simulink model "SecRwLtStHdrstFwdBkwdIsPosChk"  (R2024b)
settings: Solver=FixedStepDiscrete  StartTime=0.0  StopTime=10.0  FixedStep=0.01  RelTol=1e-3
undefined symbols (not defined in the file or in its folder): KeSMSuSecRwStHeadrestFwdBkwdPosDelta_Val, KeSMSuSecRwStHeadrestFwdBkwdPosTolr_Val
libraries: StIsPosChkLib x9, simulink x5
settings Model: Creator=sn2xws  LastModifiedBy=sn55gm
settings Model: ModifiedHistory=|
  | 2023.8.1 V2.0.0 CR401790 增加模式21-26
  | V2.1.0 ：
  | 2023.9.14 Bug 540886 修改模式判断到位的条件为10ms周期计算
  | 2023.9.15 Bug 541373Md22到位置修改为常数1代表到位置
settings SolverCC: AlgebraicLoopSolver=TrustRegion
settings DataIOCC: SaveFormat=StructureWithTime  ReturnWorkspaceOutputs=off
settings OptimizationCC: DefaultParameterBehavior=Inlined  EnhancedBackFolding=on  PassReuseOutputArgsAs=Individual arguments  ZeroExternalMemoryAtStartup=off  ZeroInternalMemoryAtStartup=off  OptimizeBlockOrder=speed  DifferentSizesBufferReuse=on  OptimizationCustomize=off  EfficientTunableParamExpr=on
settings DebuggingCC: ParameterTunabilityLossMsg=error  UnconnectedInputMsg=warning  UnconnectedOutputMsg=warning  UnconnectedLineMsg=warning  ArithmeticOperatorsInVariantConditions=warning
settings ModelReferenceCC: EnableRefExpFcnMdlSchedulingChecks=on  ModelReferenceNumInstancesAllowed=Single
settings SFSimCC: MATLABDynamicMemAlloc=off  CustomCodeUndefinedFunction=UseInterfaceOnly
settings RTWCC: Description=AUTOSAR  SystemTargetFile=autosar.tlc  GenCodeOnly=on  TemplateMakefile=ert_default_tmf  GenerateReport=on  IncludeHyperlinkInReport=on  LaunchReport=on  DataTypeReplacement=CDataTypesFixedWidth  GenerateTraceInfo=on  GenerateTraceReport=on  GenerateTraceReportSl=on  GenerateTraceReportSf=on  GenerateTraceReportEml=on  GenerateCodeMetricsReport=on  GPUComputeCapability=3.5
settings CodeAppCC: ForceParamTrailComments=on  IgnoreCustomStorageClasses=off  OperatorAnnotations=on  SimulinkDataObjDesc=on  SFDataObjDesc=on  InsertBlockDesc=on
settings STFCustomTargetCC: TargetLangStandard=C99 (ISO)  MultiwordLength=256  ParMdlRefBuildCompliant=on  CompOptLevelCompliant=on  IncludeMdlTerminateFcn=off  CombineOutputUpdateFcns=on  SuppressErrorStatus=on  ERTCustomFileBanners=on  SupportNonFinite=off  SupportComplex=off  SupportContinuousTime=off  SupportNonInlinedSFcns=off  RemoveResetFunc=on  MATLABClassNameForMDSCustomization=Simulink.SoftwareTarget.ERTCustomization  AutosarCompliant=on  UseToolchainInfoCompliant=on  LookupTableObjectStructAxisOrder=2,1,3,4,...  LUTObjectStructOrderEvenSpacing=Size,Table,Breakpoints  SystemTargetFile=autosar.tlc
settings ERTTargetCC: TargetLangStandard=C99 (ISO)  ConcurrentExecutionCompliant=off  IncludeMdlTerminateFcn=off  SuppressErrorStatus=on  SupportNonFinite=off  SupportComplex=off  ModelStepFunctionPrototypeControlCompliant=off  CPPClassGenCompliant=off  AutosarCompliant=on  LookupTableObjectStructAxisOrder=2,1,3,4,...  LUTObjectStructOrderEvenSpacing=Size,Table,Breakpoints  ERTCustomFileTemplate=example_file_process.tlc  ERTFilePackagingFormat=Compact  BooleanTrueId=TRUE  BooleanFalseId=FALSE  DynamicArrayContainerType=coder::array

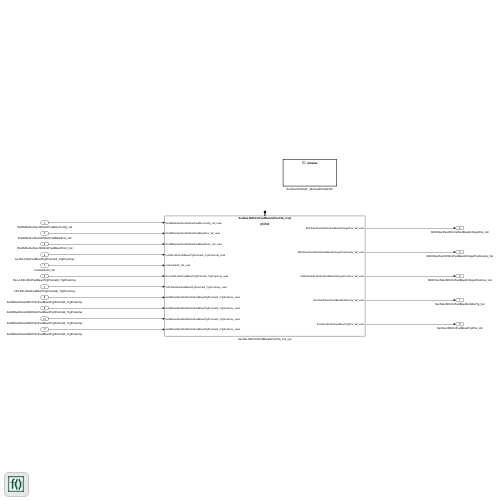
[thumbnail: Simulink's stored preview of the top-level diagram]
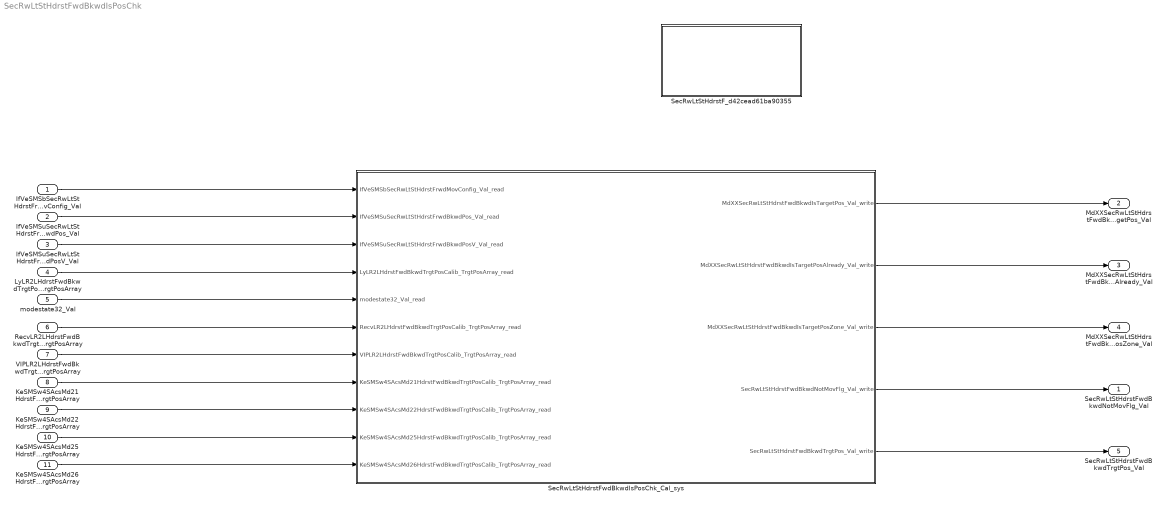
== system SecRwLtStHdrstFwdBkwdIsPosChk ==
  IfVeSMSbSecRwLtStHdrstFrwdMovConfig_Val : Inport  OutDataTypeStr=boolean  PortDimensions=1
  IfVeSMSuSecRwLtStHdrstFrwdBkwdPos_Val : Inport  Port=2  OutDataTypeStr=uint16  PortDimensions=1
  IfVeSMSuSecRwLtStHdrstFrwdBkwdPosV_Val : Inport  Port=3  OutDataTypeStr=boolean  PortDimensions=1
  LyLR2LHdrstFwdBkwdTrgtPosCalib_TrgtPosArray : Inport  Description=|  Port=4  OutDataTypeStr=uint16  PortDimensions=3
      | 0:Pos
      | 1:Max
      | 2:Min
  modestate32_Val : Inport  Port=5  OutDataTypeStr=uint32  PortDimensions=1
  RecvLR2LHdrstFwdBkwdTrgtPosCalib_TrgtPosArray : Inport  Description=|  Port=6  OutDataTypeStr=uint16  PortDimensions=3
      | 0:Pos
      | 1:Max
      | 2:Min
  VIPLR2LHdrstFwdBkwdTrgtPosCalib_TrgtPosArray : Inport  Description=|  Port=7  OutDataTypeStr=uint16  PortDimensions=3
      | 0:Pos
      | 1:Max
      | 2:Min
  KeSMSw4SAcsMd21HdrstFwdBkwdTrgtPosCalib_TrgtPosArray : Inport  Description=|  Port=8  OutDataTypeStr=uint16  PortDimensions=3
      | 0:Pos
      | 1:Max
      | 2:Min
  KeSMSw4SAcsMd22HdrstFwdBkwdTrgtPosCalib_TrgtPosArray : Inport  Description=|  Port=9  OutDataTypeStr=uint16  PortDimensions=3
      | 0:Pos
      | 1:Max
      | 2:Min
  KeSMSw4SAcsMd25HdrstFwdBkwdTrgtPosCalib_TrgtPosArray : Inport  Description=|  Port=10  OutDataTypeStr=uint16  PortDimensions=3
      | 0:Pos
      | 1:Max
      | 2:Min
  KeSMSw4SAcsMd26HdrstFwdBkwdTrgtPosCalib_TrgtPosArray : Inport  Description=|  Port=11  OutDataTypeStr=uint16  PortDimensions=3
      | 0:Pos
      | 1:Max
      | 2:Min
  SecRwLtStHdrstF_d42cead61ba90355 : Subsystem
  SecRwLtStHdrstFwdBkwdIsPosChk_Cal_sys : Subsystem
  SecRwLtStHdrstFwdBkwdNotMovFlg_Val : Outport  OutDataTypeStr=boolean  PortDimensions=1  VectorParamsAs1DForOutWhenUnconnected=off
  MdXXSecRwLtStHdrstFwdBkwdIsTargetPos_Val : Outport  Port=2  OutDataTypeStr=uint32  PortDimensions=1  VectorParamsAs1DForOutWhenUnconnected=off
  MdXXSecRwLtStHdrstFwdBkwdIsTargetPosAlready_Val : Outport  Port=3  OutDataTypeStr=uint32  PortDimensions=1  VectorParamsAs1DForOutWhenUnconnected=off
  MdXXSecRwLtStHdrstFwdBkwdIsTargetPosZone_Val : Outport  Port=4  OutDataTypeStr=uint32  PortDimensions=1  VectorParamsAs1DForOutWhenUnconnected=off
  SecRwLtStHdrstFwdBkwdTrgtPos_Val : Outport  Port=5  OutDataTypeStr=uint16  PortDimensions=1  VectorParamsAs1DForOutWhenUnconnected=off
  wires:
  IfVeSMSbSecRwLtStHdrstFrwdMovConfig_Val/1 -> SecRwLtStHdrstFwdBkwdIsPosChk_Cal_sys/1(IfVeSMSbSecRwLtStHdrstFrwdMovConfig_Val_read)
  IfVeSMSuSecRwLtStHdrstFrwdBkwdPos_Val/1 -> SecRwLtStHdrstFwdBkwdIsPosChk_Cal_sys/2(IfVeSMSuSecRwLtStHdrstFrwdBkwdPos_Val_read)
  IfVeSMSuSecRwLtStHdrstFrwdBkwdPosV_Val/1 -> SecRwLtStHdrstFwdBkwdIsPosChk_Cal_sys/3(IfVeSMSuSecRwLtStHdrstFrwdBkwdPosV_Val_read)
  LyLR2LHdrstFwdBkwdTrgtPosCalib_TrgtPosArray/1 -> SecRwLtStHdrstFwdBkwdIsPosChk_Cal_sys/4(LyLR2LHdrstFwdBkwdTrgtPosCalib_TrgtPosArray_read)
  modestate32_Val/1 -> SecRwLtStHdrstFwdBkwdIsPosChk_Cal_sys/5(modestate32_Val_read)
  RecvLR2LHdrstFwdBkwdTrgtPosCalib_TrgtPosArray/1 -> SecRwLtStHdrstFwdBkwdIsPosChk_Cal_sys/6(RecvLR2LHdrstFwdBkwdTrgtPosCalib_TrgtPosArray_read)
  VIPLR2LHdrstFwdBkwdTrgtPosCalib_TrgtPosArray/1 -> SecRwLtStHdrstFwdBkwdIsPosChk_Cal_sys/7(VIPLR2LHdrstFwdBkwdTrgtPosCalib_TrgtPosArray_read)
  SecRwLtStHdrstFwdBkwdIsPosChk_Cal_sys/1(MdXXSecRwLtStHdrstFwdBkwdIsTargetPos_Val_write) -> MdXXSecRwLtStHdrstFwdBkwdIsTargetPos_Val/1
  SecRwLtStHdrstFwdBkwdIsPosChk_Cal_sys/2(MdXXSecRwLtStHdrstFwdBkwdIsTargetPosAlready_Val_write) -> MdXXSecRwLtStHdrstFwdBkwdIsTargetPosAlready_Val/1
  SecRwLtStHdrstFwdBkwdIsPosChk_Cal_sys/3(MdXXSecRwLtStHdrstFwdBkwdIsTargetPosZone_Val_write) -> MdXXSecRwLtStHdrstFwdBkwdIsTargetPosZone_Val/1
  SecRwLtStHdrstFwdBkwdIsPosChk_Cal_sys/4(SecRwLtStHdrstFwdBkwdNotMovFlg_Val_write) -> SecRwLtStHdrstFwdBkwdNotMovFlg_Val/1
  SecRwLtStHdrstFwdBkwdIsPosChk_Cal_sys/5(SecRwLtStHdrstFwdBkwdTrgtPos_Val_write) -> SecRwLtStHdrstFwdBkwdTrgtPos_Val/1
  KeSMSw4SAcsMd21HdrstFwdBkwdTrgtPosCalib_TrgtPosArray/1 -> SecRwLtStHdrstFwdBkwdIsPosChk_Cal_sys/8(KeSMSw4SAcsMd21HdrstFwdBkwdTrgtPosCalib_TrgtPosArray_read)
  KeSMSw4SAcsMd22HdrstFwdBkwdTrgtPosCalib_TrgtPosArray/1 -> SecRwLtStHdrstFwdBkwdIsPosChk_Cal_sys/9(KeSMSw4SAcsMd22HdrstFwdBkwdTrgtPosCalib_TrgtPosArray_read)
  KeSMSw4SAcsMd25HdrstFwdBkwdTrgtPosCalib_TrgtPosArray/1 -> SecRwLtStHdrstFwdBkwdIsPosChk_Cal_sys/10(KeSMSw4SAcsMd25HdrstFwdBkwdTrgtPosCalib_TrgtPosArray_read)
  KeSMSw4SAcsMd26HdrstFwdBkwdTrgtPosCalib_TrgtPosArray/1 -> SecRwLtStHdrstFwdBkwdIsPosChk_Cal_sys/11(KeSMSw4SAcsMd26HdrstFwdBkwdTrgtPosCalib_TrgtPosArray_read)

== system SecRwLtStHdrstFwdBkwdIsPosChk/SecRwLtStHdrstF_d42cead61ba90355 ==
  note: Added blocks
  note: Added blocks
  Event Listener : EventListener  EventName=reset
  PA_KeSMSuSecRwStHeadrestFwdBkwdPosDelta_Val : Constant  Value=KeSMSuSecRwStHeadrestFwdBkwdPosDelta_Val
  PA_KeSMSuSecRwStHeadrestFwdBkwdPosTolr_Val : Constant  Value=KeSMSuSecRwStHeadrestFwdBkwdPosTolr_Val
  Terminator_1 : Terminator
  Terminator_2 : Terminator
  wires:
  PA_KeSMSuSecRwStHeadrestFwdBkwdPosDelta_Val/1 -> Terminator_1/1
  PA_KeSMSuSecRwStHeadrestFwdBkwdPosTolr_Val/1 -> Terminator_2/1

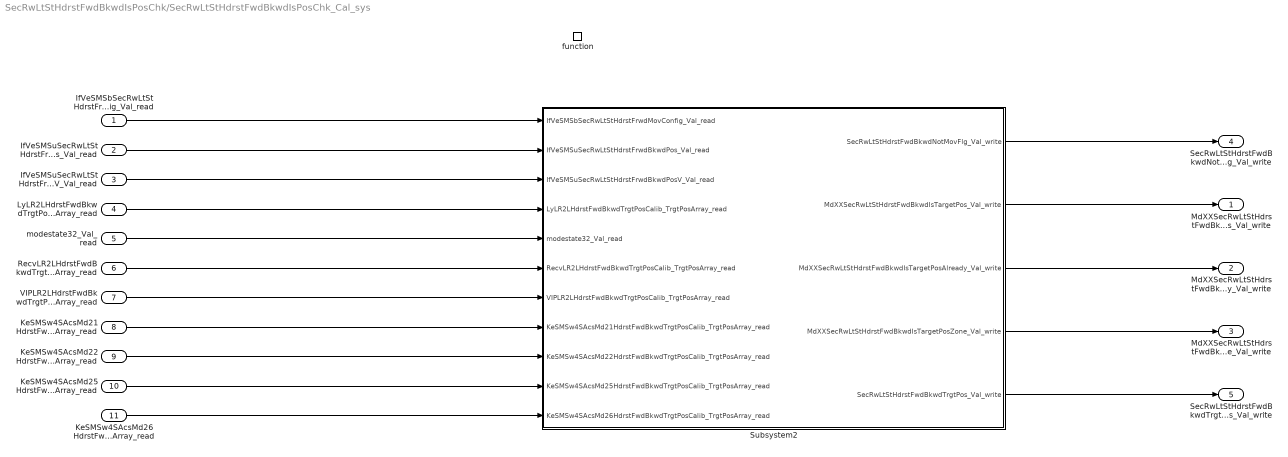
== system SecRwLtStHdrstFwdBkwdIsPosChk/SecRwLtStHdrstFwdBkwdIsPosChk_Cal_sys ==
  IfVeSMSbSecRwLtStHdrstFrwdMovConfig_Val_read : Inport
  IfVeSMSuSecRwLtStHdrstFrwdBkwdPos_Val_read : Inport  Port=2
  IfVeSMSuSecRwLtStHdrstFrwdBkwdPosV_Val_read : Inport  Port=3
  LyLR2LHdrstFwdBkwdTrgtPosCalib_TrgtPosArray_read : Inport  Port=4
  modestate32_Val_read : Inport  Port=5
  RecvLR2LHdrstFwdBkwdTrgtPosCalib_TrgtPosArray_read : Inport  Port=6
  VIPLR2LHdrstFwdBkwdTrgtPosCalib_TrgtPosArray_read : Inport  Port=7
  KeSMSw4SAcsMd21HdrstFwdBkwdTrgtPosCalib_TrgtPosArray_read : Inport  Port=8
  KeSMSw4SAcsMd22HdrstFwdBkwdTrgtPosCalib_TrgtPosArray_read : Inport  Port=9
  KeSMSw4SAcsMd25HdrstFwdBkwdTrgtPosCalib_TrgtPosArray_read : Inport  Port=10
  KeSMSw4SAcsMd26HdrstFwdBkwdTrgtPosCalib_TrgtPosArray_read : Inport  Port=11
  function : TriggerPort  TriggerType=function-call  IsSimulinkFunction=on  FunctionName=SecRwLtStHdrstFwdBkwdIsPosChk_Cal  VariantControl=(inherit)
  Subsystem2 : Subsystem
  MdXXSecRwLtStHdrstFwdBkwdIsTargetPos_Val_write : Outport  VectorParamsAs1DForOutWhenUnconnected=off
      settings: EnsureOutportIsVirtual=on
  MdXXSecRwLtStHdrstFwdBkwdIsTargetPosAlready_Val_write : Outport  Port=2  VectorParamsAs1DForOutWhenUnconnected=off
      settings: EnsureOutportIsVirtual=on
  MdXXSecRwLtStHdrstFwdBkwdIsTargetPosZone_Val_write : Outport  Port=3  VectorParamsAs1DForOutWhenUnconnected=off
      settings: EnsureOutportIsVirtual=on
  SecRwLtStHdrstFwdBkwdNotMovFlg_Val_write : Outport  Port=4  VectorParamsAs1DForOutWhenUnconnected=off
      settings: EnsureOutportIsVirtual=on
  SecRwLtStHdrstFwdBkwdTrgtPos_Val_write : Outport  Port=5  VectorParamsAs1DForOutWhenUnconnected=off
      settings: EnsureOutportIsVirtual=on
  wires:
  Subsystem2/4(MdXXSecRwLtStHdrstFwdBkwdIsTargetPosZone_Val_write) -> MdXXSecRwLtStHdrstFwdBkwdIsTargetPosZone_Val_write/1
  Subsystem2/3(MdXXSecRwLtStHdrstFwdBkwdIsTargetPosAlready_Val_write) -> MdXXSecRwLtStHdrstFwdBkwdIsTargetPosAlready_Val_write/1
  Subsystem2/1(SecRwLtStHdrstFwdBkwdNotMovFlg_Val_write) -> SecRwLtStHdrstFwdBkwdNotMovFlg_Val_write/1
  Subsystem2/2(MdXXSecRwLtStHdrstFwdBkwdIsTargetPos_Val_write) -> MdXXSecRwLtStHdrstFwdBkwdIsTargetPos_Val_write/1
  Subsystem2/5(SecRwLtStHdrstFwdBkwdTrgtPos_Val_write) -> SecRwLtStHdrstFwdBkwdTrgtPos_Val_write/1
  LyLR2LHdrstFwdBkwdTrgtPosCalib_TrgtPosArray_read/1 -> Subsystem2/4(LyLR2LHdrstFwdBkwdTrgtPosCalib_TrgtPosArray_read)
  modestate32_Val_read/1 -> Subsystem2/5(modestate32_Val_read)
  RecvLR2LHdrstFwdBkwdTrgtPosCalib_TrgtPosArray_read/1 -> Subsystem2/6(RecvLR2LHdrstFwdBkwdTrgtPosCalib_TrgtPosArray_read)
  VIPLR2LHdrstFwdBkwdTrgtPosCalib_TrgtPosArray_read/1 -> Subsystem2/7(VIPLR2LHdrstFwdBkwdTrgtPosCalib_TrgtPosArray_read)
  IfVeSMSuSecRwLtStHdrstFrwdBkwdPosV_Val_read/1 -> Subsystem2/3(IfVeSMSuSecRwLtStHdrstFrwdBkwdPosV_Val_read)
  IfVeSMSuSecRwLtStHdrstFrwdBkwdPos_Val_read/1 -> Subsystem2/2(IfVeSMSuSecRwLtStHdrstFrwdBkwdPos_Val_read)
  KeSMSw4SAcsMd21HdrstFwdBkwdTrgtPosCalib_TrgtPosArray_read/1 -> Subsystem2/8(KeSMSw4SAcsMd21HdrstFwdBkwdTrgtPosCalib_TrgtPosArray_read)
  IfVeSMSbSecRwLtStHdrstFrwdMovConfig_Val_read/1 -> Subsystem2/1(IfVeSMSbSecRwLtStHdrstFrwdMovConfig_Val_read)
  KeSMSw4SAcsMd22HdrstFwdBkwdTrgtPosCalib_TrgtPosArray_read/1 -> Subsystem2/9(KeSMSw4SAcsMd22HdrstFwdBkwdTrgtPosCalib_TrgtPosArray_read)
  KeSMSw4SAcsMd25HdrstFwdBkwdTrgtPosCalib_TrgtPosArray_read/1 -> Subsystem2/10(KeSMSw4SAcsMd25HdrstFwdBkwdTrgtPosCalib_TrgtPosArray_read)
  KeSMSw4SAcsMd26HdrstFwdBkwdTrgtPosCalib_TrgtPosArray_read/1 -> Subsystem2/11(KeSMSw4SAcsMd26HdrstFwdBkwdTrgtPosCalib_TrgtPosArray_read)

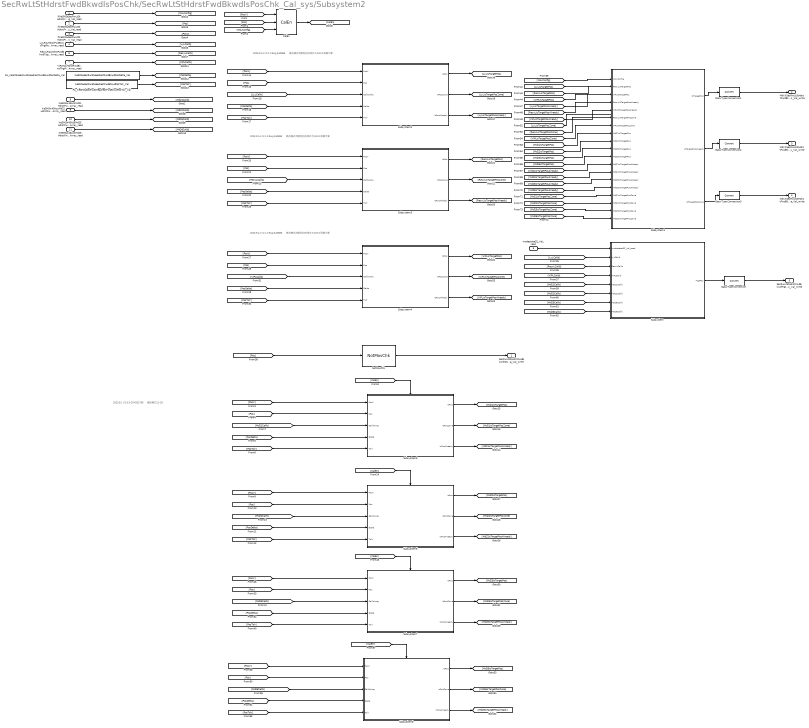
== system SecRwLtStHdrstFwdBkwdIsPosChk/SecRwLtStHdrstFwdBkwdIsPosChk_Cal_sys/Subsystem2 ==
  note: 2023.9.14 V2.1.0 Bug 540886 修改模式判断到位的条件为10ms周期计算
  note: 2023.9.14 V2.1.0 Bug 540886 修改模式判断到位的条件为10ms周期计算
  note: 2023.9.14 V2.1.0 Bug 540886 修改模式判断到位的条件为10ms周期计算
  note: 2023.8.1 V2.0.0 CR4201790 增加模式21-26
  IfVeSMSbSecRwLtStHdrstFrwdMovConfig_Val_read : Inport
  IfVeSMSuSecRwLtStHdrstFrwdBkwdPos_Val_read : Inport  Port=2
  IfVeSMSuSecRwLtStHdrstFrwdBkwdPosV_Val_read : Inport  Port=3
  LyLR2LHdrstFwdBkwdTrgtPosCalib_TrgtPosArray_read : Inport  Port=4
  modestate32_Val_read : Inport  Port=5
  RecvLR2LHdrstFwdBkwdTrgtPosCalib_TrgtPosArray_read : Inport  Port=6
  VIPLR2LHdrstFwdBkwdTrgtPosCalib_TrgtPosArray_read : Inport  Port=7
  KeSMSw4SAcsMd21HdrstFwdBkwdTrgtPosCalib_TrgtPosArray_read : Inport  Port=8
  KeSMSw4SAcsMd22HdrstFwdBkwdTrgtPosCalib_TrgtPosArray_read : Inport  Port=9
  KeSMSw4SAcsMd25HdrstFwdBkwdTrgtPosCalib_TrgtPosArray_read : Inport  Port=10
  KeSMSw4SAcsMd26HdrstFwdBkwdTrgtPosCalib_TrgtPosArray_read : Inport  Port=11
  CalEn : StIsPosChkLib/CalEn  SystemSampleTime=-1  VariantActivationTime=update diagram  AllowFlexibleInterface=on  Latency=0  AutoFrameSizeCalculation=off
  Data Type Conversion{,1..3} (4 alike) : DataTypeConversion  SaturateOnIntegerOverflow=off  RndMeth=Floor
  NotMovChk : StIsPosChkLib/NotMovChk  SystemSampleTime=-1  VariantActivationTime=update diagram  AllowFlexibleInterface=on  Latency=0  AutoFrameSizeCalculation=off
  PA_KeSMSuSecRwStHeadrestFwdBkwdPosDelta_Val : Constant  Value=KeSMSuSecRwStHeadrestFwdBkwdPosDelta_Val
  PA_KeSMSuSecRwStHeadrestFwdBkwdPosTolr_Val : Constant  Value=KeSMSuSecRwStHeadrestFwdBkwdPosTolr_Val
  Subsystem : Subsystem
  Subsystem1 : Subsystem
  Subsystem2 : Subsystem
  Subsystem3 : Subsystem
  Subsystem4 : Subsystem
  Subsystem5 : Subsystem
  Subsystem6 : Subsystem
  Subsystem7 : Subsystem
  Subsystem8 : Subsystem
  SecRwLtStHdrstFwdBkwdNotMovFlg_Val_write : Outport  VectorParamsAs1DForOutWhenUnconnected=off
      settings: EnsureOutportIsVirtual=on
  MdXXSecRwLtStHdrstFwdBkwdIsTargetPos_Val_write : Outport  Port=2  VectorParamsAs1DForOutWhenUnconnected=off
      settings: EnsureOutportIsVirtual=on
  MdXXSecRwLtStHdrstFwdBkwdIsTargetPosAlready_Val_write : Outport  Port=3  VectorParamsAs1DForOutWhenUnconnected=off
      settings: EnsureOutportIsVirtual=on
  MdXXSecRwLtStHdrstFwdBkwdIsTargetPosZone_Val_write : Outport  Port=4  VectorParamsAs1DForOutWhenUnconnected=off
      settings: EnsureOutportIsVirtual=on
  SecRwLtStHdrstFwdBkwdTrgtPos_Val_write : Outport  Port=5  VectorParamsAs1DForOutWhenUnconnected=off
      settings: EnsureOutportIsVirtual=on
  wires:
  CalEn/1 -> [CalEn]
  IfVeSMSuSecRwLtStHdrstFrwdBkwdPosV_Val_read/1 -> [PosV]
  Subsystem4/2(IsPosZone) -> [VIPLIsTargetPosZone]
  Subsystem2/3(IsPosAlready) -> [LyLIsTargetPosAlready]
  [PosDelta] -> Subsystem2/4(Delta)
  NotMovChk/1 -> SecRwLtStHdrstFwdBkwdNotMovFlg_Val_write/1
  PA_KeSMSuSecRwStHeadrestFwdBkwdPosDelta_Val/1 -> [PosDelta]
  Data Type Conversion3/1 -> MdXXSecRwLtStHdrstFwdBkwdIsTargetPosZone_Val_write/1
  [Pos] -> CalEn/2
  [Pos] -> NotMovChk/1
  [VIPLCalib] -> Subsystem4/3(CalibArray)
  Subsystem4/3(IsPosAlready) -> [VIPLIsTargetPosAlready]
  [PosTolr] -> Subsystem2/5(Tolr)
  Data Type Conversion2/1 -> MdXXSecRwLtStHdrstFwdBkwdIsTargetPosAlready_Val_write/1
  [Pos] -> Subsystem3/2(Pos)
  modestate32_Val_read/1 -> Subsystem/1(modestate32_Val_read)
  Subsystem4/1(IsPos) -> [VIPLIsTargetPos]
  [RecvLCalib] -> Subsystem3/3(CalibArray)
  RecvLR2LHdrstFwdBkwdTrgtPosCalib_TrgtPosArray_read/1 -> [RecvLCalib]
  [LyLCalib] -> Subsystem/2(LyLCalib)
  Subsystem/1(TrgtPos) -> Data Type Conversion/1
  Subsystem3/3(IsPosAlready) -> [RecvLIsTargetPosAlready]
  [Pos] -> Subsystem4/2(Pos)
  Subsystem3/2(IsPosZone) -> [RecvLIsTargetPosZone]
  [PosV] -> Subsystem4/1(PosV)
  IfVeSMSuSecRwLtStHdrstFrwdBkwdPos_Val_read/1 -> [Pos]
  Subsystem1/3(IsTargetPosZone) -> Data Type Conversion3/1
  [PosV] -> Subsystem2/1(PosV)
  Subsystem3/1(IsPos) -> [RecvLIsTargetPos]
  Subsystem2/1(IsPos) -> [LyLIsTargetPos]
  [PosTolr] -> Subsystem4/5(Tolr)
  [MovConfig] -> Subsystem1/1(MovConfig)
  Subsystem2/2(IsPosZone) -> [LyLIsTargetPosZone]
  [PosV] -> Subsystem3/1(PosV)
  [LyLIsTargetPos] -> ?
  [PosTolr] -> Subsystem3/5(Tolr)
  Subsystem1/2(IsTargetPosAlready) -> Data Type Conversion2/1
  [LyLIsTargetPosZone] -> ?
  [Pos] -> Subsystem2/2(Pos)
  [PosV] -> CalEn/1
  IfVeSMSbSecRwLtStHdrstFrwdMovConfig_Val_read/1 -> [MovConfig]
  [RecvLIsTargetPosAlready] -> Subsystem1/4(RecvLIsTargetPosAlready)
  [PosDelta] -> Subsystem4/4(Delta)
  [PosDelta] -> Subsystem3/4(Delta)
  Subsystem1/1(IsTargetPos) -> Data Type Conversion1/1
  PA_KeSMSuSecRwStHeadrestFwdBkwdPosTolr_Val/1 -> [PosTolr]
  [MovConfig] -> CalEn/3
  [RecvLCalib] -> Subsystem/3(RecvLCalib)
  Data Type Conversion/1 -> SecRwLtStHdrstFwdBkwdTrgtPos_Val_write/1
  [RecvLIsTargetPos] -> Subsystem1/2(RecvLIsTargetPos)
  [VIPLIsTargetPos] -> Subsystem1/3(VIPLIsTargetPos)
  [LyLCalib] -> Subsystem2/3(CalibArray)
  [VIPLIsTargetPosZone] -> Subsystem1/7(VIPLIsTargetPosZone)
  [LyLIsTargetPosAlready] -> ?
  Data Type Conversion1/1 -> MdXXSecRwLtStHdrstFwdBkwdIsTargetPos_Val_write/1
  [VIPLCalib] -> Subsystem/4(VIPLCalib)
  [RecvLIsTargetPosZone] -> Subsystem1/6(RecvLIsTargetPosZone)
  [VIPLIsTargetPosAlready] -> Subsystem1/5(VIPLIsTargetPosAlready)
  LyLR2LHdrstFwdBkwdTrgtPosCalib_TrgtPosArray_read/1 -> [LyLCalib]
  VIPLR2LHdrstFwdBkwdTrgtPosCalib_TrgtPosArray_read/1 -> [VIPLCalib]
  KeSMSw4SAcsMd21HdrstFwdBkwdTrgtPosCalib_TrgtPosArray_read/1 -> [Md21Calib]
  KeSMSw4SAcsMd22HdrstFwdBkwdTrgtPosCalib_TrgtPosArray_read/1 -> [Md22Calib]
  KeSMSw4SAcsMd25HdrstFwdBkwdTrgtPosCalib_TrgtPosArray_read/1 -> [Md25Calib]
  KeSMSw4SAcsMd26HdrstFwdBkwdTrgtPosCalib_TrgtPosArray_read/1 -> [Md26Calib]
  [PosDelta] -> Subsystem5/4(Delta)
  [CalEn] -> Subsystem5/Enable
  [PosTolr] -> Subsystem5/5(Tolr)
  [PosV] -> Subsystem5/1(PosV)
  [Pos] -> Subsystem5/2(Pos)
  Subsystem5/1(IsPos) -> [Md21IsTargetPos]
  Subsystem5/3(IsPosAlready) -> [Md21IsTargetPosAlready]
  [Md21Calib] -> Subsystem5/3(CalibArray)
  Subsystem5/2(IsPosZone) -> [Md21IsTargetPosZone]
  Subsystem6/2(IsPosZone) -> [Md22IsTargetPosZone]
  [Md22Calib] -> Subsystem6/3(CalibArray)
  Subsystem6/3(IsPosAlready) -> [Md22IsTargetPosAlready]
  Subsystem6/1(IsPos) -> [Md22IsTargetPos]
  [Pos] -> Subsystem6/2(Pos)
  [PosV] -> Subsystem6/1(PosV)
  [PosTolr] -> Subsystem6/5(Tolr)
  [CalEn] -> Subsystem6/Enable
  [PosDelta] -> Subsystem6/4(Delta)
  [PosDelta] -> Subsystem7/4(Delta)
  [CalEn] -> Subsystem7/Enable
  [PosTolr] -> Subsystem7/5(Tolr)
  [PosV] -> Subsystem7/1(PosV)
  [Pos] -> Subsystem7/2(Pos)
  Subsystem7/1(IsPos) -> [Md25IsTargetPos]
  Subsystem7/3(IsPosAlready) -> [Md25IsTargetPosAlready]
  [Md25Calib] -> Subsystem7/3(CalibArray)
  Subsystem7/2(IsPosZone) -> [Md25IsTargetPosZone]
  Subsystem8/2(IsPosZone) -> [Md26IsTargetPosZone]
  [Md26Calib] -> Subsystem8/3(CalibArray)
  Subsystem8/3(IsPosAlready) -> [Md26IsTargetPosAlready]
  Subsystem8/1(IsPos) -> [Md26IsTargetPos]
  [Pos] -> Subsystem8/2(Pos)
  [PosV] -> Subsystem8/1(PosV)
  [PosTolr] -> Subsystem8/5(Tolr)
  [CalEn] -> Subsystem8/Enable
  [PosDelta] -> Subsystem8/4(Delta)
  [Md21Calib] -> Subsystem/5(Md21Calib)
  [Md22Calib] -> Subsystem/6(Md22Calib)
  [Md25Calib] -> Subsystem/7(Md25Calib)
  [Md26Calib] -> Subsystem/8(Md26Calib)
  [Md21IsTargetPos] -> Subsystem1/8(Md21IsTargetPos)
  [Md22IsTargetPos] -> Subsystem1/9(Md22IsTargetPos)
  [Md25IsTargetPos] -> Subsystem1/10(Md25IsTargetPos)
  [Md26IsTargetPos] -> Subsystem1/11(Md26IsTargetPos)
  [Md21IsTargetPosAlready] -> Subsystem1/12(Md21IsTargetPosAlready)
  [Md22IsTargetPosAlready] -> Subsystem1/13(Md22IsTargetPosAlready)
  [Md25IsTargetPosAlready] -> Subsystem1/14(Md25IsTargetPosAlready)
  [Md26IsTargetPosAlready] -> Subsystem1/15(Md26IsTargetPosAlready)
  [Md21IsTargetPosZone] -> Subsystem1/16(Md21IsTargetPosZone)
  [Md22IsTargetPosZone] -> Subsystem1/17(Md22IsTargetPosZone)
  [Md25IsTargetPosZone] -> Subsystem1/18(Md25IsTargetPosZone)
  [Md26IsTargetPosZone] -> Subsystem1/19(Md26IsTargetPosZone)

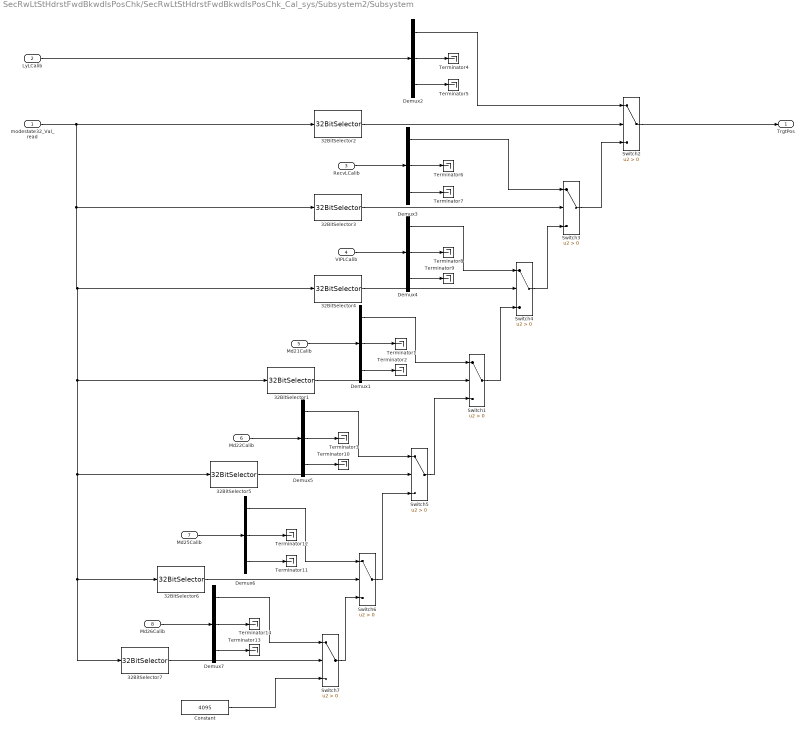
== system SecRwLtStHdrstFwdBkwdIsPosChk/SecRwLtStHdrstFwdBkwdIsPosChk_Cal_sys/Subsystem2/Subsystem ==
  modestate32_Val_read : Inport
  LyLCalib : Inport  Port=2
  RecvLCalib : Inport  Port=3
  VIPLCalib : Inport  Port=4
  Md21Calib : Inport  Port=5
  Md22Calib : Inport  Port=6
  Md25Calib : Inport  Port=7
  Md26Calib : Inport  Port=8
  32BitSelector1 : StIsPosChkLib/32BitSelector  BitNum=20
  32BitSelector2 : StIsPosChkLib/32BitSelector  BitNum=13
  32BitSelector3 : StIsPosChkLib/32BitSelector  BitNum=10
  32BitSelector4 : StIsPosChkLib/32BitSelector  BitNum=9
  32BitSelector5 : StIsPosChkLib/32BitSelector  BitNum=21
  32BitSelector6 : StIsPosChkLib/32BitSelector  BitNum=24
  32BitSelector7 : StIsPosChkLib/32BitSelector  BitNum=25
  Constant : Constant  Value=4095  OutDataTypeStr=uint16
  Demux{1..7} (7 alike) : Demux  Outputs=3
  Switch{1..7} (7 alike) : Switch  Criteria=u2 > Threshold  SaturateOnIntegerOverflow=off  InputSameDT=off
  Terminator{1..14} (14 alike) : Terminator
  TrgtPos : Outport  VectorParamsAs1DForOutWhenUnconnected=off
      settings: EnsureOutportIsVirtual=on
  wires:
  Switch2/1 -> TrgtPos/1
  Switch3/1 -> Switch2/3
  Switch4/1 -> Switch3/3
  32BitSelector2/1 -> Switch2/2
  32BitSelector3/1 -> Switch3/2
  32BitSelector4/1 -> Switch4/2
  Demux2/1 -> Switch2/1
  Demux2/3 -> Terminator5/1
  Demux2/2 -> Terminator4/1
  LyLCalib/1 -> Demux2/1
  RecvLCalib/1 -> Demux3/1
  Demux3/2 -> Terminator6/1
  Demux3/3 -> Terminator7/1
  Demux3/1 -> Switch3/1
  Demux4/1 -> Switch4/1
  Demux4/3 -> Terminator9/1
  Demux4/2 -> Terminator8/1
  VIPLCalib/1 -> Demux4/1
  Md21Calib/1 -> Demux1/1
  Demux1/2 -> Terminator1/1
  Demux1/3 -> Terminator2/1
  Demux1/1 -> Switch1/1
  32BitSelector1/1 -> Switch1/2
  Switch5/1 -> Switch1/3
  Switch6/1 -> Switch5/3
  32BitSelector5/1 -> Switch5/2
  Demux5/1 -> Switch5/1
  Demux5/3 -> Terminator10/1
  Demux5/2 -> Terminator3/1
  Md22Calib/1 -> Demux5/1
  Md25Calib/1 -> Demux6/1
  Demux6/2 -> Terminator12/1
  Demux6/3 -> Terminator11/1
  Demux6/1 -> Switch6/1
  32BitSelector6/1 -> Switch6/2
  Switch7/1 -> Switch6/3
  modestate32_Val_read/1 -> 32BitSelector2/1, 32BitSelector3/1, 32BitSelector7/1, 32BitSelector6/1, 32BitSelector5/1, 32BitSelector1/1, 32BitSelector4/1
  Constant/1 -> Switch7/3
  32BitSelector7/1 -> Switch7/2
  Demux7/1 -> Switch7/1
  Demux7/3 -> Terminator13/1
  Demux7/2 -> Terminator14/1
  Md26Calib/1 -> Demux7/1
  Switch1/1 -> Switch4/3

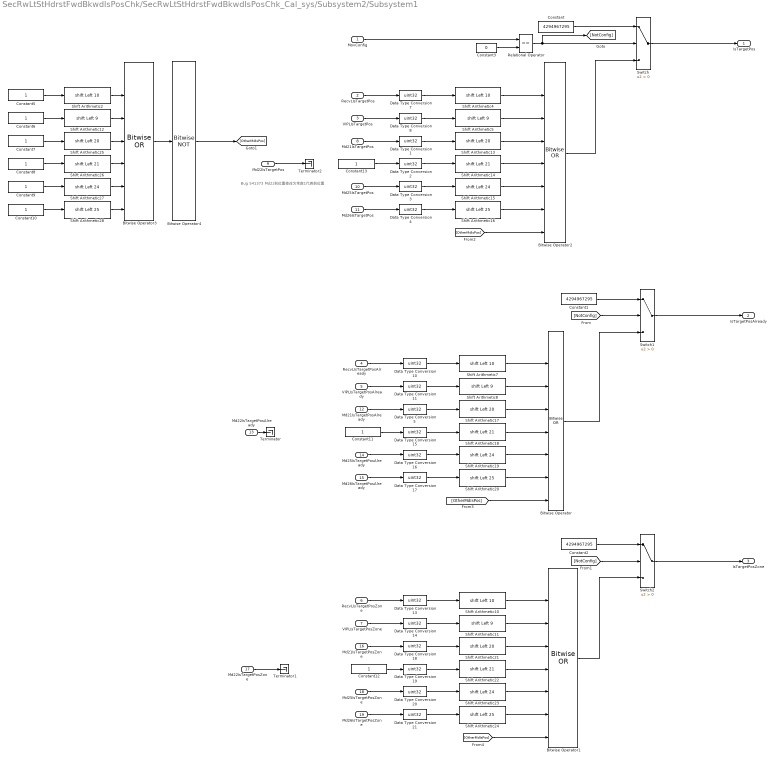
== system SecRwLtStHdrstFwdBkwdIsPosChk/SecRwLtStHdrstFwdBkwdIsPosChk_Cal_sys/Subsystem2/Subsystem1 ==
  note: Bug 541373 Md22到位置修改为常数1代表到位置
  MovConfig : Inport
  RecvLIsTargetPos : Inport  Port=2
  VIPLIsTargetPos : Inport  Port=3
  RecvLIsTargetPosAlready : Inport  Port=4
  VIPLIsTargetPosAlready : Inport  Port=5
  RecvLIsTargetPosZone : Inport  Port=6
  VIPLIsTargetPosZone : Inport  Port=7
  Md21IsTargetPos : Inport  Port=8
  Md22IsTargetPos : Inport  Port=9
  Md25IsTargetPos : Inport  Port=10
  Md26IsTargetPos : Inport  Port=11
  Md21IsTargetPosAlready : Inport  Port=12
  Md22IsTargetPosAlready : Inport  Port=13
  Md25IsTargetPosAlready : Inport  Port=14
  Md26IsTargetPosAlready : Inport  Port=15
  Md21IsTargetPosZone : Inport  Port=16
  Md22IsTargetPosZone : Inport  Port=17
  Md25IsTargetPosZone : Inport  Port=18
  Md26IsTargetPosZone : Inport  Port=19
  Bitwise Operator : simulink/Logic and Bit Operations/Bitwise Operator  logicop=OR  UseBitMask=off  NumInputPorts=8  BitMask=bin2dec('11011001')  BitMaskRealWorld=Stored Integer
  Bitwise Operator1 : simulink/Logic and Bit Operations/Bitwise Operator  logicop=OR  UseBitMask=off  NumInputPorts=8  BitMask=bin2dec('11011001')  BitMaskRealWorld=Stored Integer
  Bitwise Operator2 : simulink/Logic and Bit Operations/Bitwise Operator  logicop=OR  UseBitMask=off  NumInputPorts=8  BitMask=bin2dec('11011001')  BitMaskRealWorld=Stored Integer
  Bitwise Operator3 : simulink/Logic and Bit Operations/Bitwise Operator  logicop=OR  UseBitMask=off  NumInputPorts=7  BitMask=bin2dec('11011001')  BitMaskRealWorld=Stored Integer
  Bitwise Operator4 : simulink/Logic and Bit Operations/Bitwise Operator  logicop=NOT  UseBitMask=off  BitMask=bin2dec('11011001')  BitMaskRealWorld=Stored Integer
  Constant : Constant  Value=4294967295  OutDataTypeStr=uint32
  Constant1 : Constant  Value=4294967295  OutDataTypeStr=uint32
  Constant{5..13} (9 alike) : Constant  OutDataTypeStr=uint32
  Constant2 : Constant  Value=4294967295  OutDataTypeStr=uint32
  Constant3 : Constant  Value=0  OutDataTypeStr=uint8
  Data Type Conversion{1..5,7..8,10..11,13..21} (18 alike) : DataTypeConversion  OutDataTypeStr=uint32  SaturateOnIntegerOverflow=off  RndMeth=Floor
  Relational Operator : RelationalOperator  Operator===  OutDataTypeStr=boolean  RndMeth=Simplest  InputSameDT=off
  Shift Arithmetic{2,4,7,10} (4 alike) : ArithShift  BitShiftNumber=10  BitShiftDirection=Left
  Shift Arithmetic{5,8,11..12} (4 alike) : ArithShift  BitShiftNumber=9  BitShiftDirection=Left
  Shift Arithmetic{13,17,21,25} (4 alike) : ArithShift  BitShiftNumber=20  BitShiftDirection=Left
  Shift Arithmetic{14,18,22,26} (4 alike) : ArithShift  BitShiftNumber=21  BitShiftDirection=Left
  Shift Arithmetic{15,19,23,27} (4 alike) : ArithShift  BitShiftNumber=24  BitShiftDirection=Left
  Shift Arithmetic{16,20,24,28} (4 alike) : ArithShift  BitShiftNumber=25  BitShiftDirection=Left
  Switch : Switch  Criteria=u2 > Threshold  SaturateOnIntegerOverflow=off  InputSameDT=off
  Switch1 : Switch  Criteria=u2 > Threshold  SaturateOnIntegerOverflow=off  InputSameDT=off
  Switch2 : Switch  Criteria=u2 > Threshold  SaturateOnIntegerOverflow=off  InputSameDT=off
  Terminator : Terminator
  Terminator1 : Terminator
  Terminator2 : Terminator
  IsTargetPos : Outport  VectorParamsAs1DForOutWhenUnconnected=off
      settings: EnsureOutportIsVirtual=on
  IsTargetPosAlready : Outport  Port=2  VectorParamsAs1DForOutWhenUnconnected=off
      settings: EnsureOutportIsVirtual=on
  IsTargetPosZone : Outport  Port=3  VectorParamsAs1DForOutWhenUnconnected=off
      settings: EnsureOutportIsVirtual=on
  wires:
  Constant3/1 -> Relational Operator/2
  Constant/1 -> Switch/1
  Relational Operator/1 -> [NotConfig], Switch/2
  MovConfig/1 -> Relational Operator/1
  Switch/1 -> IsTargetPos/1
  [NotConfig] -> Switch1/2
  Constant1/1 -> Switch1/1
  Switch1/1 -> IsTargetPosAlready/1
  Switch2/1 -> IsTargetPosZone/1
  Constant2/1 -> Switch2/1
  [NotConfig] -> Switch2/2
  Bitwise Operator1/1 -> Switch2/3
  Bitwise Operator/1 -> Switch1/3
  Bitwise Operator2/1 -> Switch/3
  Shift Arithmetic4/1 -> Bitwise Operator2/2
  Shift Arithmetic5/1 -> Bitwise Operator2/3
  Data Type Conversion7/1 -> Shift Arithmetic4/1
  Data Type Conversion8/1 -> Shift Arithmetic5/1
  RecvLIsTargetPos/1 -> Data Type Conversion7/1
  VIPLIsTargetPos/1 -> Data Type Conversion8/1
  VIPLIsTargetPosAlready/1 -> Data Type Conversion11/1
  RecvLIsTargetPosAlready/1 -> Data Type Conversion10/1
  Data Type Conversion11/1 -> Shift Arithmetic8/1
  Data Type Conversion10/1 -> Shift Arithmetic7/1
  Shift Arithmetic8/1 -> Bitwise Operator/3
  Shift Arithmetic7/1 -> Bitwise Operator/2
  Data Type Conversion14/1 -> Shift Arithmetic11/1
  Data Type Conversion13/1 -> Shift Arithmetic10/1
  VIPLIsTargetPosZone/1 -> Data Type Conversion14/1
  Shift Arithmetic10/1 -> Bitwise Operator1/2
  RecvLIsTargetPosZone/1 -> Data Type Conversion13/1
  Shift Arithmetic11/1 -> Bitwise Operator1/3
  Shift Arithmetic2/1 -> Bitwise Operator3/2
  Constant5/1 -> Shift Arithmetic2/1
  Shift Arithmetic12/1 -> Bitwise Operator3/3
  Constant6/1 -> Shift Arithmetic12/1
  Bitwise Operator3/1 -> Bitwise Operator4/1
  Bitwise Operator4/1 -> [OtherMdIsPos]
  [OtherMdIsPos] -> Bitwise Operator2/8
  [OtherMdIsPos] -> Bitwise Operator/8
  Md21IsTargetPos/1 -> Data Type Conversion1/1
  Data Type Conversion1/1 -> Shift Arithmetic13/1
  Shift Arithmetic13/1 -> Bitwise Operator2/4
  Shift Arithmetic14/1 -> Bitwise Operator2/5
  Data Type Conversion2/1 -> Shift Arithmetic14/1
  Md25IsTargetPos/1 -> Data Type Conversion3/1
  Data Type Conversion3/1 -> Shift Arithmetic15/1
  Shift Arithmetic15/1 -> Bitwise Operator2/6
  Shift Arithmetic16/1 -> Bitwise Operator2/7
  Data Type Conversion4/1 -> Shift Arithmetic16/1
  Md26IsTargetPos/1 -> Data Type Conversion4/1
  [OtherMdIsPos] -> Bitwise Operator1/8
  Md25IsTargetPosAlready/1 -> Data Type Conversion16/1
  Shift Arithmetic19/1 -> Bitwise Operator/6
  Data Type Conversion16/1 -> Shift Arithmetic19/1
  Md26IsTargetPosAlready/1 -> Data Type Conversion17/1
  Md21IsTargetPosAlready/1 -> Data Type Conversion5/1
  Shift Arithmetic20/1 -> Bitwise Operator/7
  Shift Arithmetic18/1 -> Bitwise Operator/5
  Data Type Conversion5/1 -> Shift Arithmetic17/1
  Shift Arithmetic17/1 -> Bitwise Operator/4
  Data Type Conversion17/1 -> Shift Arithmetic20/1
  Data Type Conversion15/1 -> Shift Arithmetic18/1
  Md25IsTargetPosZone/1 -> Data Type Conversion20/1
  Shift Arithmetic23/1 -> Bitwise Operator1/6
  Data Type Conversion20/1 -> Shift Arithmetic23/1
  Md26IsTargetPosZone/1 -> Data Type Conversion21/1
  Md21IsTargetPosZone/1 -> Data Type Conversion18/1
  Shift Arithmetic24/1 -> Bitwise Operator1/7
  Shift Arithmetic22/1 -> Bitwise Operator1/5
  Data Type Conversion18/1 -> Shift Arithmetic21/1
  Shift Arithmetic21/1 -> Bitwise Operator1/4
  Data Type Conversion21/1 -> Shift Arithmetic24/1
  Data Type Conversion19/1 -> Shift Arithmetic22/1
  Constant7/1 -> Shift Arithmetic25/1
  Constant8/1 -> Shift Arithmetic26/1
  Constant9/1 -> Shift Arithmetic27/1
  Shift Arithmetic27/1 -> Bitwise Operator3/6
  Constant10/1 -> Shift Arithmetic28/1
  Shift Arithmetic25/1 -> Bitwise Operator3/4
  Shift Arithmetic26/1 -> Bitwise Operator3/5
  Shift Arithmetic28/1 -> Bitwise Operator3/7
  Md22IsTargetPosAlready/1 -> Terminator/1
  Constant11/1 -> Data Type Conversion15/1
  Constant12/1 -> Data Type Conversion19/1
  Md22IsTargetPosZone/1 -> Terminator1/1
  Constant13/1 -> Data Type Conversion2/1
  Md22IsTargetPos/1 -> Terminator2/1

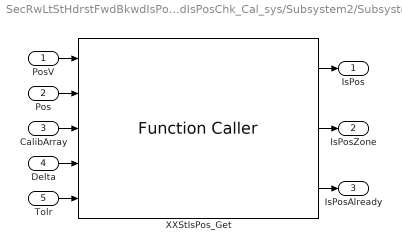
== system SecRwLtStHdrstFwdBkwdIsPosChk/SecRwLtStHdrstFwdBkwdIsPosChk_Cal_sys/Subsystem2/Subsystem2 ==
  PosV : Inport
  Pos : Inport  Port=2
  CalibArray : Inport  Port=3
  Delta : Inport  Port=4
  Tolr : Inport  Port=5
  XXStIsPos_Get : FunctionCaller  FunctionPrototype=[IsPos,IsPosZone,IsPosAlready] = XXStIsPos_Get(PosV,Pos,CalibArray,Delta,Tolr)  InputArgumentSpecifications=boolean(true), uint16(1), uint16([1;1;1]), uint16(1), uint16(1)  OutputArgumentSpecifications=boolean(true), boolean(true), boolean(true)
  IsPos : Outport  VectorParamsAs1DForOutWhenUnconnected=off
  IsPosZone : Outport  Port=2  VectorParamsAs1DForOutWhenUnconnected=off
  IsPosAlready : Outport  Port=3  VectorParamsAs1DForOutWhenUnconnected=off
  wires:
  Pos/1 -> XXStIsPos_Get/2
  Delta/1 -> XXStIsPos_Get/4
  PosV/1 -> XXStIsPos_Get/1
  CalibArray/1 -> XXStIsPos_Get/3
  XXStIsPos_Get/2 -> IsPosZone/1
  XXStIsPos_Get/1 -> IsPos/1
  XXStIsPos_Get/3 -> IsPosAlready/1
  Tolr/1 -> XXStIsPos_Get/5

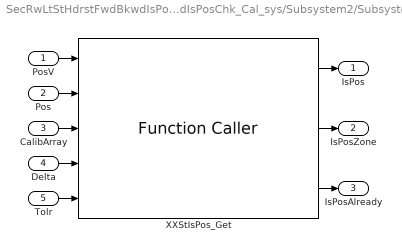
== system SecRwLtStHdrstFwdBkwdIsPosChk/SecRwLtStHdrstFwdBkwdIsPosChk_Cal_sys/Subsystem2/Subsystem3 ==
  PosV : Inport
  Pos : Inport  Port=2
  CalibArray : Inport  Port=3
  Delta : Inport  Port=4
  Tolr : Inport  Port=5
  XXStIsPos_Get : FunctionCaller  FunctionPrototype=[IsPos,IsPosZone,IsPosAlready] = XXStIsPos_Get(PosV,Pos,CalibArray,Delta,Tolr)  InputArgumentSpecifications=boolean(true), uint16(1), uint16([1;1;1]), uint16(1), uint16(1)  OutputArgumentSpecifications=boolean(true), boolean(true), boolean(true)
  IsPos : Outport  VectorParamsAs1DForOutWhenUnconnected=off
  IsPosZone : Outport  Port=2  VectorParamsAs1DForOutWhenUnconnected=off
  IsPosAlready : Outport  Port=3  VectorParamsAs1DForOutWhenUnconnected=off
  wires:
  Pos/1 -> XXStIsPos_Get/2
  Delta/1 -> XXStIsPos_Get/4
  PosV/1 -> XXStIsPos_Get/1
  CalibArray/1 -> XXStIsPos_Get/3
  XXStIsPos_Get/2 -> IsPosZone/1
  XXStIsPos_Get/1 -> IsPos/1
  XXStIsPos_Get/3 -> IsPosAlready/1
  Tolr/1 -> XXStIsPos_Get/5

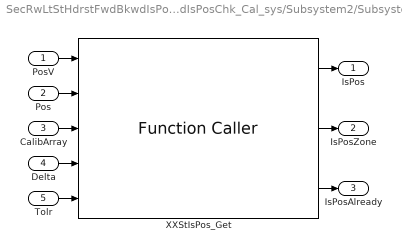
== system SecRwLtStHdrstFwdBkwdIsPosChk/SecRwLtStHdrstFwdBkwdIsPosChk_Cal_sys/Subsystem2/Subsystem4 ==
  PosV : Inport
  Pos : Inport  Port=2
  CalibArray : Inport  Port=3
  Delta : Inport  Port=4
  Tolr : Inport  Port=5
  XXStIsPos_Get : FunctionCaller  FunctionPrototype=[IsPos,IsPosZone,IsPosAlready] = XXStIsPos_Get(PosV,Pos,CalibArray,Delta,Tolr)  InputArgumentSpecifications=boolean(true), uint16(1), uint16([1;1;1]), uint16(1), uint16(1)  OutputArgumentSpecifications=boolean(true), boolean(true), boolean(true)
  IsPos : Outport  VectorParamsAs1DForOutWhenUnconnected=off
  IsPosZone : Outport  Port=2  VectorParamsAs1DForOutWhenUnconnected=off
  IsPosAlready : Outport  Port=3  VectorParamsAs1DForOutWhenUnconnected=off
  wires:
  Pos/1 -> XXStIsPos_Get/2
  Delta/1 -> XXStIsPos_Get/4
  PosV/1 -> XXStIsPos_Get/1
  CalibArray/1 -> XXStIsPos_Get/3
  XXStIsPos_Get/2 -> IsPosZone/1
  XXStIsPos_Get/1 -> IsPos/1
  XXStIsPos_Get/3 -> IsPosAlready/1
  Tolr/1 -> XXStIsPos_Get/5

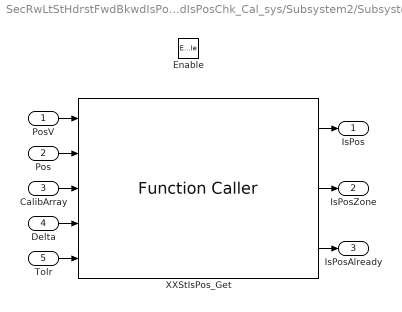
== system SecRwLtStHdrstFwdBkwdIsPosChk/SecRwLtStHdrstFwdBkwdIsPosChk_Cal_sys/Subsystem2/Subsystem5 ==
  PosV : Inport
  Pos : Inport  Port=2
  CalibArray : Inport  Port=3
  Delta : Inport  Port=4
  Tolr : Inport  Port=5
  Enable : EnablePort
  XXStIsPos_Get : FunctionCaller  FunctionPrototype=[IsPos,IsPosZone,IsPosAlready] = XXStIsPos_Get(PosV,Pos,CalibArray,Delta,Tolr)  InputArgumentSpecifications=boolean(true), uint16(1), uint16([1;1;1]), uint16(1), uint16(1)  OutputArgumentSpecifications=boolean(true), boolean(true), boolean(true)
  IsPos : Outport  VectorParamsAs1DForOutWhenUnconnected=off
  IsPosZone : Outport  Port=2  VectorParamsAs1DForOutWhenUnconnected=off
  IsPosAlready : Outport  Port=3  VectorParamsAs1DForOutWhenUnconnected=off
  wires:
  Tolr/1 -> XXStIsPos_Get/5
  XXStIsPos_Get/3 -> IsPosAlready/1
  XXStIsPos_Get/1 -> IsPos/1
  XXStIsPos_Get/2 -> IsPosZone/1
  CalibArray/1 -> XXStIsPos_Get/3
  PosV/1 -> XXStIsPos_Get/1
  Delta/1 -> XXStIsPos_Get/4
  Pos/1 -> XXStIsPos_Get/2

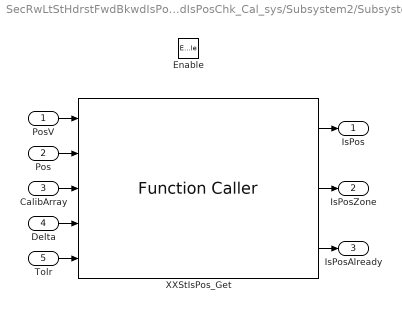
== system SecRwLtStHdrstFwdBkwdIsPosChk/SecRwLtStHdrstFwdBkwdIsPosChk_Cal_sys/Subsystem2/Subsystem6 ==
  PosV : Inport
  Pos : Inport  Port=2
  CalibArray : Inport  Port=3
  Delta : Inport  Port=4
  Tolr : Inport  Port=5
  Enable : EnablePort
  XXStIsPos_Get : FunctionCaller  FunctionPrototype=[IsPos,IsPosZone,IsPosAlready] = XXStIsPos_Get(PosV,Pos,CalibArray,Delta,Tolr)  InputArgumentSpecifications=boolean(true), uint16(1), uint16([1;1;1]), uint16(1), uint16(1)  OutputArgumentSpecifications=boolean(true), boolean(true), boolean(true)
  IsPos : Outport  VectorParamsAs1DForOutWhenUnconnected=off
  IsPosZone : Outport  Port=2  VectorParamsAs1DForOutWhenUnconnected=off
  IsPosAlready : Outport  Port=3  VectorParamsAs1DForOutWhenUnconnected=off
  wires:
  Pos/1 -> XXStIsPos_Get/2
  Delta/1 -> XXStIsPos_Get/4
  PosV/1 -> XXStIsPos_Get/1
  CalibArray/1 -> XXStIsPos_Get/3
  XXStIsPos_Get/2 -> IsPosZone/1
  XXStIsPos_Get/1 -> IsPos/1
  XXStIsPos_Get/3 -> IsPosAlready/1
  Tolr/1 -> XXStIsPos_Get/5

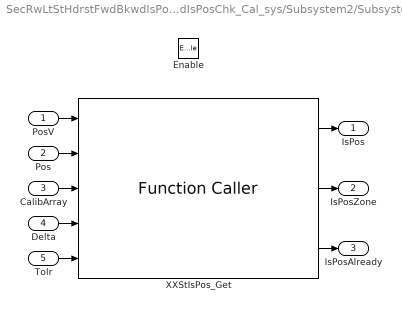
== system SecRwLtStHdrstFwdBkwdIsPosChk/SecRwLtStHdrstFwdBkwdIsPosChk_Cal_sys/Subsystem2/Subsystem7 ==
  PosV : Inport
  Pos : Inport  Port=2
  CalibArray : Inport  Port=3
  Delta : Inport  Port=4
  Tolr : Inport  Port=5
  Enable : EnablePort
  XXStIsPos_Get : FunctionCaller  FunctionPrototype=[IsPos,IsPosZone,IsPosAlready] = XXStIsPos_Get(PosV,Pos,CalibArray,Delta,Tolr)  InputArgumentSpecifications=boolean(true), uint16(1), uint16([1;1;1]), uint16(1), uint16(1)  OutputArgumentSpecifications=boolean(true), boolean(true), boolean(true)
  IsPos : Outport  VectorParamsAs1DForOutWhenUnconnected=off
  IsPosZone : Outport  Port=2  VectorParamsAs1DForOutWhenUnconnected=off
  IsPosAlready : Outport  Port=3  VectorParamsAs1DForOutWhenUnconnected=off
  wires:
  Tolr/1 -> XXStIsPos_Get/5
  XXStIsPos_Get/3 -> IsPosAlready/1
  XXStIsPos_Get/1 -> IsPos/1
  XXStIsPos_Get/2 -> IsPosZone/1
  CalibArray/1 -> XXStIsPos_Get/3
  PosV/1 -> XXStIsPos_Get/1
  Delta/1 -> XXStIsPos_Get/4
  Pos/1 -> XXStIsPos_Get/2

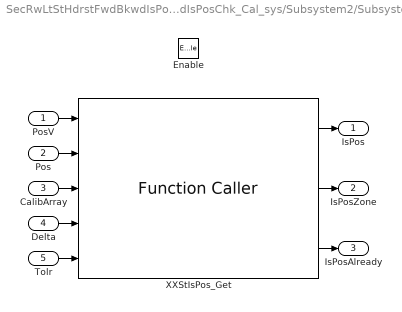
== system SecRwLtStHdrstFwdBkwdIsPosChk/SecRwLtStHdrstFwdBkwdIsPosChk_Cal_sys/Subsystem2/Subsystem8 ==
  PosV : Inport
  Pos : Inport  Port=2
  CalibArray : Inport  Port=3
  Delta : Inport  Port=4
  Tolr : Inport  Port=5
  Enable : EnablePort
  XXStIsPos_Get : FunctionCaller  FunctionPrototype=[IsPos,IsPosZone,IsPosAlready] = XXStIsPos_Get(PosV,Pos,CalibArray,Delta,Tolr)  InputArgumentSpecifications=boolean(true), uint16(1), uint16([1;1;1]), uint16(1), uint16(1)  OutputArgumentSpecifications=boolean(true), boolean(true), boolean(true)
  IsPos : Outport  VectorParamsAs1DForOutWhenUnconnected=off
  IsPosZone : Outport  Port=2  VectorParamsAs1DForOutWhenUnconnected=off
  IsPosAlready : Outport  Port=3  VectorParamsAs1DForOutWhenUnconnected=off
  wires:
  Pos/1 -> XXStIsPos_Get/2
  Delta/1 -> XXStIsPos_Get/4
  PosV/1 -> XXStIsPos_Get/1
  CalibArray/1 -> XXStIsPos_Get/3
  XXStIsPos_Get/2 -> IsPosZone/1
  XXStIsPos_Get/1 -> IsPos/1
  XXStIsPos_Get/3 -> IsPosAlready/1
  Tolr/1 -> XXStIsPos_Get/5
